simulink model "PEMFC_cEGR_Core_Physical_v01"  (R2025b)
settings: Solver=VariableStepAuto  StartTime=0.0  StopTime=500  RelTol=1e-3
PreLoadFcn:
  | addpath('D:\matlab2025b\toolbox\physmod\fluids\supporting_files\example_libraries'); addpath('E:\agentwork_pemfc_cEGR_0519\04_Simulink物理网络模型\02_参数'); P_pemfc_cEGR = PEMFC_cEGR_params_v01();
InitFcn:
  | addpath('D:\matlab2025b\toolbox\physmod\fluids\supporting_files\example_libraries'); addpath('E:\agentwork_pemfc_cEGR_0519\04_Simulink物理网络模型\02_参数'); P_pemfc_cEGR = PEMFC_cEGR_params_v01();
undefined symbols (not defined in the file): P_pemfc_cEGR
libraries: FuelCell_lib x17, nesl_utility x13, fl_lib x8
(part 1 of 3)
settings Model: Creator=ADMIN  LastModifiedBy=ADMIN

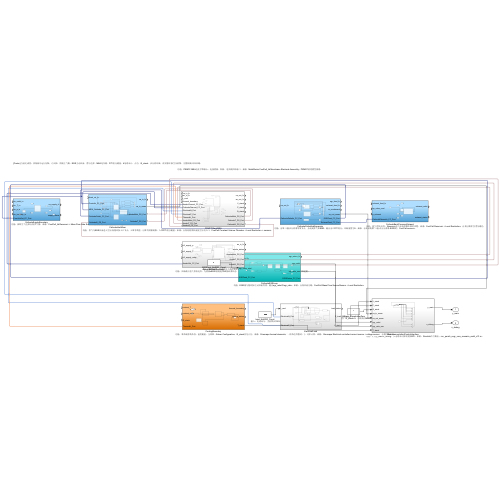
[thumbnail: Simulink's stored preview of the top-level diagram]
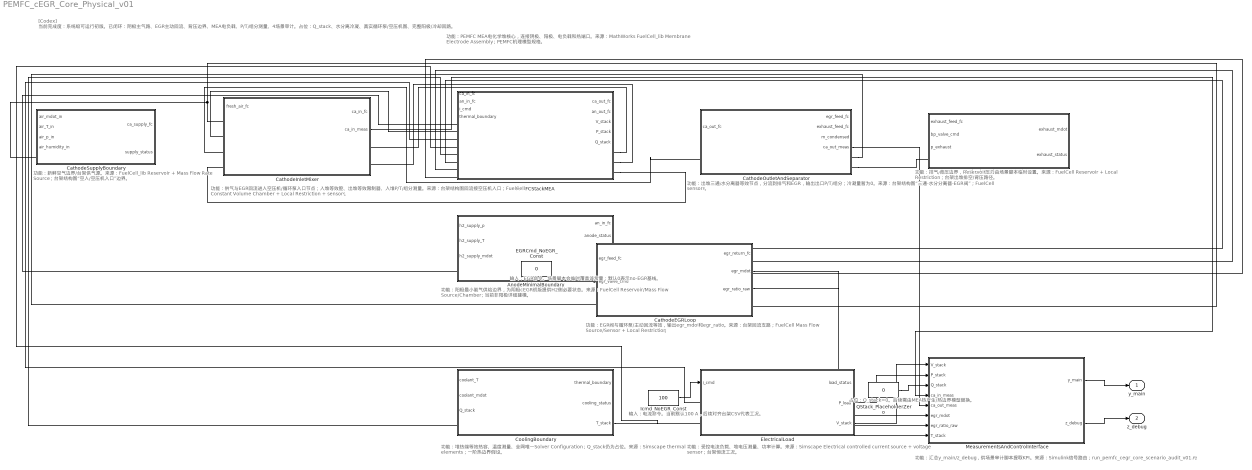
== system PEMFC_cEGR_Core_Physical_v01 ==
  note: [Codex] 当前完成度：系统级可运行初版。已闭环：阴极主气路、EGR主动回流、背压边界、MEA电负载、P/T/组分测量、4场景审计。占位：Q_stack、水分离冷凝、真实循环泵/空压机图、完整阳极/冷却回路。
  note: 功能：新鲜空气边界/台架供气源。来源：FuelCell_lib Reservoir + Mass Flow Rate Source；台架结构图“空入/空压机入口”边界。
  note: 功能：供气与EGR回流进入空压机/循环泵入口节点；入堆等效腔、出堆等效限制器、入堆P/T/组分测量。来源：台架结构图回流接空压机入口；FuelCell Constant Volume Chamber + Local Restriction + sensors。
  note: 功能：PEMFC MEA电化学堆核心，连接阴极、阳极、电负载和热端口。来源：MathWorks FuelCell_lib Membrane Electrode Assembly；PEMFC机理模型规格。
  note: 功能：出堆三通/水分离器等效节点，分流到排气和EGR，输出出口P/T/组分；冷凝量暂为0。来源：台架结构图“三通-水分分离器-EGR阀”；FuelCell sensors。
  note: 功能：排气/背压边界，Reservoir压力由场景脚本临时设置。来源：FuelCell Reservoir + Local Restriction；台架出堆排空/背压路径。
  note: 功能：EGR阀与循环泵/主动回流等效，输出egr_mdot和egr_ratio。来源：台架回流支路；FuelCell Mass Flow Source/Sensor + Local Restriction。
  note: 功能：阳极最小氢气供给边界，为阴极cEGR初版提供H2侧必要状态。来源：FuelCell Reservoir/Mass Flow Source/Chamber；当前非阳极详细建模。
  note: 功能：堆热端等效热容、温度测量、全网唯一Solver Configuration；Q_stack仍为占位。来源：Simscape thermal elements；一阶热边界假设。
  note: 功能：受控电流负载、堆电压测量、功率计算。来源：Simscape Electrical controlled current source + voltage sensor；台架恒流工况。
  note: 功能：汇总y_main/z_debug，供场景审计脚本提取KPI。来源：Simulink信号路由；run_pemfc_cegr_core_scenario_audit_v01.m。
  note: 输入：EGR命令。场景脚本会临时覆盖该常量；默认0表示no-EGR基线。
  note: 输入：电流命令。当前默认100 A，后续对齐台架CSV代表工况。
  note: 占位：Q_stack=0。后续需由MEA热产生/热边界模型替换。
  AnodeMinimalBoundary : Subsystem
  CathodeBackPressureExhaust : Subsystem
  CathodeEGRLoop : Subsystem
  CathodeInletMixer : Subsystem
  CathodeOutletAndSeparator : Subsystem
  CathodeSupplyBoundary : Subsystem
  CoolingBoundary : Subsystem
  EGRCmd_NoEGR_Const : Constant  Value=0
  ElectricalLoad : Subsystem
  Icmd_NoEGR_Const : Constant  Value=100
  MeasurementsAndControlInterface : Subsystem
  PEMFCStackMEA : Subsystem
  QStack_PlaceholderZero : Constant  Value=0
  y_main : Outport
  z_debug : Outport  Port=2
  wires:
  Icmd_NoEGR_Const/1 -> ElectricalLoad/1(i_cmd)
  EGRCmd_NoEGR_Const/1 -> CathodeEGRLoop/2(egr_valve_cmd)
  ElectricalLoad/3(V_stack) -> MeasurementsAndControlInterface/1(V_stack)
  ElectricalLoad/2(P_load) -> MeasurementsAndControlInterface/2(P_stack)
  QStack_PlaceholderZero/1 -> MeasurementsAndControlInterface/3(Q_stack)
  CathodeEGRLoop/2(egr_mdot) -> MeasurementsAndControlInterface/6(egr_mdot)
  CathodeEGRLoop/3(egr_ratio_raw) -> MeasurementsAndControlInterface/7(egr_ratio_raw)
  MeasurementsAndControlInterface/1(y_main) -> y_main/1
  MeasurementsAndControlInterface/2(z_debug) -> z_debug/1
  CathodeInletMixer/2(ca_in_meas) -> MeasurementsAndControlInterface/4(ca_in_meas)
  CathodeOutletAndSeparator/4(ca_out_meas) -> MeasurementsAndControlInterface/5(ca_out_meas)
  CoolingBoundary/3(T_stack) -> MeasurementsAndControlInterface/8(T_stack)
  connections:
  AnodeMinimalBoundary/LConn1 -- PEMFCStackMEA/LConn1
  CathodeInletMixer/LConn2 -- PEMFCStackMEA/LConn2
  CathodeSupplyBoundary/LConn1 -- CathodeInletMixer/LConn1 -- CathodeEGRLoop/RConn1
  PEMFCStackMEA/RConn1 -- CathodeInletMixer/RConn1
  PEMFCStackMEA/RConn2 -- CathodeInletMixer/RConn2
  PEMFCStackMEA/RConn3 -- CathodeInletMixer/LConn4
  PEMFCStackMEA/LConn3 -- ElectricalLoad/LConn1
  PEMFCStackMEA/LConn4 -- ElectricalLoad/LConn2
  PEMFCStackMEA/LConn5 -- CoolingBoundary/LConn1
  AnodeMinimalBoundary/RConn1 -- PEMFCStackMEA/LConn6
  AnodeMinimalBoundary/RConn2 -- PEMFCStackMEA/LConn7
  AnodeMinimalBoundary/RConn3 -- PEMFCStackMEA/LConn8
  CathodeInletMixer/LConn3 -- CathodeOutletAndSeparator/LConn1
  CathodeOutletAndSeparator/RConn1 -- CathodeEGRLoop/LConn1
  CathodeOutletAndSeparator/RConn2 -- CathodeBackPressureExhaust/LConn1

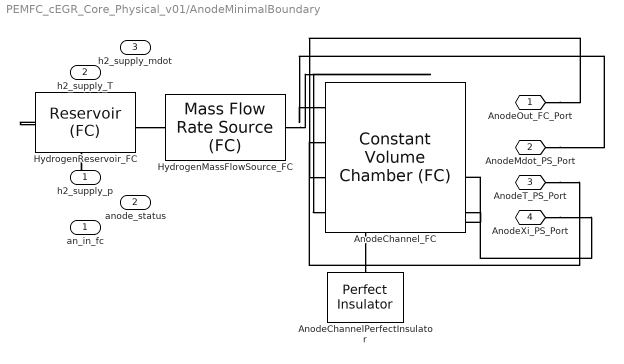
== system PEMFC_cEGR_Core_Physical_v01/AnodeMinimalBoundary ==
  h2_supply_p : Inport
  h2_supply_T : Inport  Port=2
  h2_supply_mdot : Inport  Port=3
  AnodeChannelPerfectInsulator : fl_lib/Thermal/Thermal Elements/Perfect Insulator  T_specify=off  T_priority=None  T=293.15 K  T_nominal_specify=off  T_nominal_value=1  T_nominal_unit=K
  AnodeChannel_FC : FuelCell_lib/elements/Constant Volume Chamber (FC)  V0=P_pemfc_cEGR.anode.channel_volume_m3 m^3  num_ports=foundation.enum.num_ports.two  area_A=0.01 m^2  area_B=0.01 m^2  area_C=0.01 m^2  area_D=0.01 m^2  cond_spec=FuelCell.enum.ChamberCondSpec.Enabled  tau_c=1 s  is_cond=[0; 0; 0; 0]  out_comp=FuelCell.enum.Composition.Mole  p0=P_pemfc_cEGR.anode.h2_supply_pressure_Pa Pa  T0=P_pemfc_cEGR.anode.h2_supply_temperature_K K  comp=FuelCell.enum.Composition.Mole  y0=[0; 0; 0.98; 0.02]  x0=[0; 0; 0.98; 0.02]
      settings: InternalSimscapePortConfiguration="{\"Bottom\":[{\"id\":\"H\",\"label\":\"H\",\"type\":\"foundation.thermal.thermal\"}],\"Left\":[{\"id\":\"MIn\",\"label\":\"MIn\",\"type\":\"input\"},{\"id\":\"TIn\",\"label\":\"TIn\",\"type\":\"input\"}],\"Right\":[{\"id\":\"pC\",\"label\":\"p\",\"type\":\"output\"},{\"id\":\"TC\",\"label\":\"T\",\"type\":\"output\"},{\"id\":\"yC_i\",\"label\":\"y_i\",\"type\":\"output\"}],\"Top\":[{\"id\":\"A\",\"label\":\"A\",\"type\":\"FuelCell.FuelCell\"},{\"id\":\"B\",\"label\":\"B\",\"type\":\"FuelCell.FuelCell\"}]}"
  HydrogenMassFlowSource_FC : FuelCell_lib/sources/Mass Flow Rate Source (FC)  source_type=foundation.enum.constant_controlled.constant  flow_rate=P_pemfc_cEGR.anode.h2_supply_mdot_kg_s kg/s  power_spec=foundation.enum.power_spec.none  area_A=0.01 m^2  area_B=0.01 m^2  mdot_A_specify=off  mdot_A_priority=None  mdot_A=0.1 kg/s  mdot_A_nominal_specify=off  mdot_A_nominal_value=1  mdot_A_nominal_unit=kg/s  mdot_B_specify=off  mdot_B_priority=None  mdot_B=0.1 kg/s  mdot_B_nominal_specify=off  mdot_B_nominal_value=1  mdot_B_nominal_unit=kg/s  phi_A_specify=off  phi_A_priority=None  phi_A=0 J/s  phi_A_nominal_specify=off  phi_A_nominal_value=1  phi_A_nominal_unit=J/s  phi_B_specify=off  phi_B_priority=None  phi_B=0 J/s  phi_B_nominal_specify=off  phi_B_nominal_value=1  phi_B_nominal_unit=J/s  mdot_A_i_specify=off  mdot_A_i_priority=None  mdot_A_i=[0; 0; 0; 0] kg/s  mdot_A_i_nominal_specify=off  mdot_A_i_nominal_value=1  mdot_A_i_nominal_unit=kg/s  mdot_B_i_specify=off  mdot_B_i_priority=None  mdot_B_i=[0; 0; 0; 0] kg/s  mdot_B_i_nominal_specify=off  mdot_B_i_nominal_value=1  mdot_B_i_nominal_unit=kg/s
      settings: InternalSimscapePortConfiguration="{\"Bottom\":[],\"Left\":[{\"id\":\"A\",\"label\":\"A\",\"type\":\"FuelCell.FuelCell\"}],\"Right\":[{\"id\":\"B\",\"label\":\"B\",\"type\":\"FuelCell.FuelCell\"}],\"Top\":[]}"
  HydrogenReservoir_FC : FuelCell_lib/elements/Reservoir (FC)  constCond=true  p0=P_pemfc_cEGR.anode.h2_supply_pressure_Pa Pa  T0=P_pemfc_cEGR.anode.h2_supply_temperature_K K  comp=FuelCell.enum.Composition.Mole  y0=[0; 0; 1; 0]  x0=[0; 0; 1; 0]  area=0.01 m^2
      settings: InternalSimscapePortConfiguration="{\"Bottom\":[],\"Left\":[],\"Right\":[],\"Top\":[{\"id\":\"A\",\"label\":\"A\",\"type\":\"FuelCell.FuelCell\"}]}"
  AnodeOut_FC_Port : PMIOPort  Side=Left
  AnodeMdot_PS_Port : PMIOPort  Port=2  Side=Right
  AnodeT_PS_Port : PMIOPort  Port=3  Side=Right
  AnodeXi_PS_Port : PMIOPort  Port=4  Side=Right
  an_in_fc : Outport
  anode_status : Outport  Port=2
  connections:
  AnodeMdot_PS_Port/RConn1 -- AnodeChannel_FC/LConn1
  AnodeT_PS_Port/RConn1 -- AnodeChannel_FC/LConn2
  AnodeXi_PS_Port/RConn1 -- AnodeChannel_FC/RConn3
  HydrogenReservoir_FC/LConn1 -- HydrogenMassFlowSource_FC/LConn1
  HydrogenMassFlowSource_FC/RConn1 -- AnodeChannel_FC/LConn4
  AnodeChannel_FC/RConn4 -- AnodeChannelPerfectInsulator/LConn1
  AnodeOut_FC_Port/RConn1 -- AnodeChannel_FC/LConn3

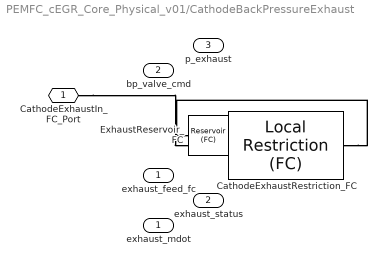
== system PEMFC_cEGR_Core_Physical_v01/CathodeBackPressureExhaust ==
  exhaust_feed_fc : Inport
  bp_valve_cmd : Inport  Port=2
  p_exhaust : Inport  Port=3
  CathodeExhaustRestriction_FC : FuelCell_lib/elements/Local Restriction (FC)  const_area=true  restriction_area=P_pemfc_cEGR.exhaust.A_max_m2 m^2  min_area=1e-10 m^2  max_area=0.005 m^2  area=0.01 m^2  Cd=P_pemfc_cEGR.exhaust.Cd  B_lam=0.999
      settings: InternalSimscapePortConfiguration="{\"Bottom\":[],\"Left\":[{\"id\":\"A\",\"label\":\"A\",\"type\":\"FuelCell.FuelCell\"}],\"Right\":[{\"id\":\"B\",\"label\":\"B\",\"type\":\"FuelCell.FuelCell\"}],\"Top\":[]}"
  ExhaustReservoir_FC : FuelCell_lib/elements/Reservoir (FC)  constCond=true  p0=P_pemfc_cEGR.active.p_exhaust_Pa Pa  T0=P_pemfc_cEGR.cathode.initial_temperature_K K  comp=FuelCell.enum.Composition.Mole  y0=[0.77; 0.21; 0; 0.02]  x0=[0.75; 0.23; 0; 0.02]  area=0.01 m^2
      settings: InternalSimscapePortConfiguration="{\"Bottom\":[],\"Left\":[],\"Right\":[],\"Top\":[{\"id\":\"A\",\"label\":\"A\",\"type\":\"FuelCell.FuelCell\"}]}"
  CathodeExhaustIn_FC_Port : PMIOPort  Side=Left
  exhaust_mdot : Outport
  exhaust_status : Outport  Port=2
  connections:
  CathodeExhaustIn_FC_Port/RConn1 -- CathodeExhaustRestriction_FC/LConn1
  CathodeExhaustRestriction_FC/RConn1 -- ExhaustReservoir_FC/LConn1

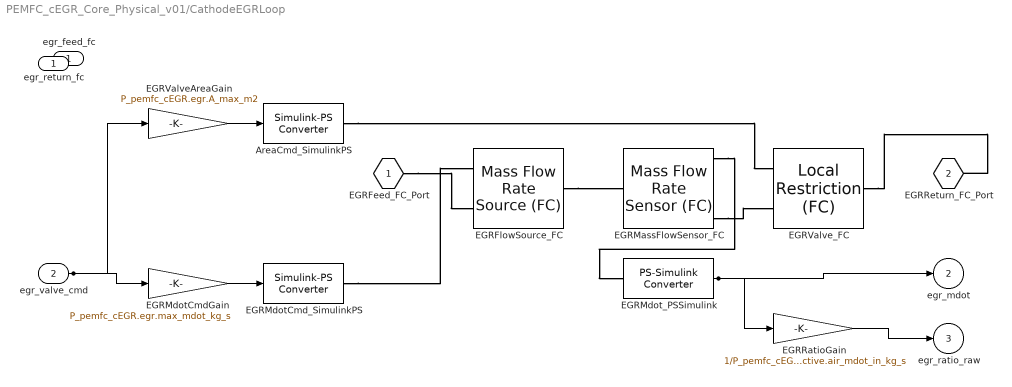
== system PEMFC_cEGR_Core_Physical_v01/CathodeEGRLoop ==
  egr_feed_fc : Inport
  egr_valve_cmd : Inport  Port=2
  AreaCmd_SimulinkPS : nesl_utility/Simulink-PS Converter  PhysicalDomain=network_engine_domain  SubClassName=ps_input  LeftPortType=input  RightPortType=output  PseudoPeriodic=off  Frequencies=[]  NoiseDistribution=none  NoiseParameters=[]  Unit=1  AffineConversion=off  FilteringAndDerivatives=provide  SimscapeFilterOrder=1  InputFilterTimeConstant=0.001  UdotUserProvided=0
  EGRFlowSource_FC : FuelCell_lib/sources/Mass Flow Rate Source (FC)  source_type=foundation.enum.constant_controlled.controlled  flow_rate=0 kg/s  power_spec=foundation.enum.power_spec.none  area_A=0.01 m^2  area_B=0.01 m^2  mdot_A_specify=off  mdot_A_priority=None  mdot_A=0.1 kg/s  mdot_A_nominal_specify=off  mdot_A_nominal_value=1  mdot_A_nominal_unit=kg/s  mdot_B_specify=off  mdot_B_priority=None  mdot_B=0.1 kg/s  mdot_B_nominal_specify=off  mdot_B_nominal_value=1  mdot_B_nominal_unit=kg/s  phi_A_specify=off  phi_A_priority=None  phi_A=0 J/s  phi_A_nominal_specify=off  phi_A_nominal_value=1  phi_A_nominal_unit=J/s  phi_B_specify=off  phi_B_priority=None  phi_B=0 J/s  phi_B_nominal_specify=off  phi_B_nominal_value=1  phi_B_nominal_unit=J/s  mdot_A_i_specify=off  mdot_A_i_priority=None  mdot_A_i=[0; 0; 0; 0] kg/s  mdot_A_i_nominal_specify=off  mdot_A_i_nominal_value=1  mdot_A_i_nominal_unit=kg/s  mdot_B_i_specify=off  mdot_B_i_priority=None  mdot_B_i=[0; 0; 0; 0] kg/s  mdot_B_i_nominal_specify=off  mdot_B_i_nominal_value=1  mdot_B_i_nominal_unit=kg/s
      settings: InternalSimscapePortConfiguration="{\"Bottom\":[],\"Left\":[{\"id\":\"M\",\"label\":\"M\",\"type\":\"input\"},{\"id\":\"A\",\"label\":\"A\",\"type\":\"FuelCell.FuelCell\"}],\"Right\":[{\"id\":\"B\",\"label\":\"B\",\"type\":\"FuelCell.FuelCell\"}],\"Top\":[]}"
  EGRMassFlowSensor_FC : FuelCell_lib/sensors/Mass Flow Rate Sensor (FC)
      settings: InternalSimscapePortConfiguration="{\"Bottom\":[],\"Left\":[{\"id\":\"A\",\"label\":\"A\",\"type\":\"FuelCell.FuelCell\"}],\"Right\":[{\"id\":\"M\",\"label\":\"M\",\"type\":\"output\"},{\"id\":\"Phi_out\",\"label\":\"Phi\",\"type\":\"output\"},{\"id\":\"M_i\",\"label\":\"M_i\",\"type\":\"output\"},{\"id\":\"B\",\"label\":\"B\",\"type\":\"FuelCell.FuelCell\"}],\"Top\":[]}"
  EGRMdotCmdGain : Gain  Gain=P_pemfc_cEGR.egr.max_mdot_kg_s
  EGRMdotCmd_SimulinkPS : nesl_utility/Simulink-PS Converter  PhysicalDomain=network_engine_domain  SubClassName=ps_input  LeftPortType=input  RightPortType=output  PseudoPeriodic=off  Frequencies=[]  NoiseDistribution=none  NoiseParameters=[]  Unit=1  AffineConversion=off  FilteringAndDerivatives=provide  SimscapeFilterOrder=1  InputFilterTimeConstant=0.001  UdotUserProvided=0
  EGRMdot_PSSimulink : nesl_utility/PS-Simulink Converter  PhysicalDomain=network_engine_domain  SubClassName=ps_output  LeftPortType=input  RightPortType=output  PseudoPeriodic=off  Frequencies=[]  VectorFormat=inherit  Unit=inherit  AffineConversion=off
  EGRRatioGain : Gain  Gain=1/P_pemfc_cEGR.active.air_mdot_in_kg_s
  EGRValveAreaGain : Gain  Gain=P_pemfc_cEGR.egr.A_max_m2
  EGRValve_FC : FuelCell_lib/elements/Local Restriction (FC)  const_area=false  restriction_area=0.001 m^2  min_area=P_pemfc_cEGR.egr.A_min_m2 m^2  max_area=P_pemfc_cEGR.egr.A_max_m2 m^2  area=0.01 m^2  Cd=P_pemfc_cEGR.egr.Cd  B_lam=0.999
      settings: InternalSimscapePortConfiguration="{\"Bottom\":[],\"Left\":[{\"id\":\"AR\",\"label\":\"AR\",\"type\":\"input\"},{\"id\":\"A\",\"label\":\"A\",\"type\":\"FuelCell.FuelCell\"}],\"Right\":[{\"id\":\"B\",\"label\":\"B\",\"type\":\"FuelCell.FuelCell\"}],\"Top\":[]}"
  EGRFeed_FC_Port : PMIOPort  Side=Left
  EGRReturn_FC_Port : PMIOPort  Port=2  Side=Right
  egr_return_fc : Outport
  egr_mdot : Outport  Port=2
  egr_ratio_raw : Outport  Port=3
  wires:
  egr_valve_cmd/1 -> EGRValveAreaGain/1, EGRMdotCmdGain/1
  EGRValveAreaGain/1 -> AreaCmd_SimulinkPS/1
  EGRMdot_PSSimulink/1 -> egr_mdot/1, EGRRatioGain/1
  EGRRatioGain/1 -> egr_ratio_raw/1
  EGRMdotCmdGain/1 -> EGRMdotCmd_SimulinkPS/1
  connections:
  AreaCmd_SimulinkPS/RConn1 -- EGRValve_FC/LConn1
  EGRMassFlowSensor_FC/RConn1 -- EGRMdot_PSSimulink/LConn1
  EGRMdotCmd_SimulinkPS/RConn1 -- EGRFlowSource_FC/LConn1
  EGRFeed_FC_Port/RConn1 -- EGRFlowSource_FC/LConn2
  EGRFlowSource_FC/RConn1 -- EGRMassFlowSensor_FC/LConn1
  EGRMassFlowSensor_FC/RConn4 -- EGRValve_FC/LConn2
  EGRValve_FC/RConn1 -- EGRReturn_FC_Port/RConn1
